simulink model "controller_main"  (R2025a)
settings: Solver=VariableStepAuto  StartTime=0.0  StopTime=inf  RelTol=1e-3
model workspace (MAT data in the model file):
  input_force = 1000
  input_moment = 300
  input_radius = 1
  input_theta = 0.785398163397
settings Model: Creator=TAK  LastModifiedBy=TAK

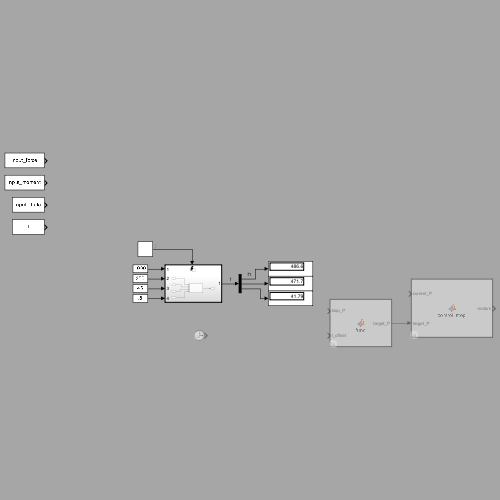
[thumbnail: Simulink's stored preview of the top-level diagram]
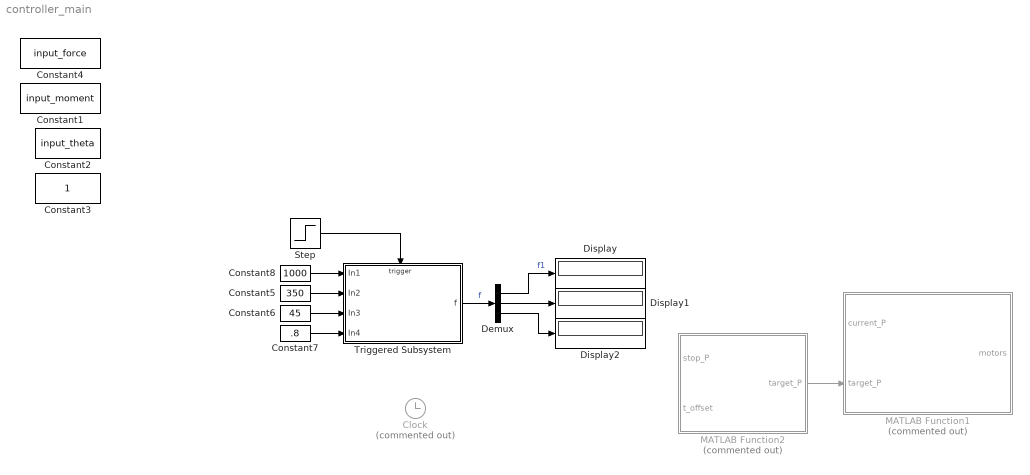
== system controller_main ==
  Clock : Clock  Commented=on
  Constant1 : Constant  Value=input_moment
  Constant2 : Constant  Value=input_theta
  Constant3 : Constant
  Constant4 : Constant  Value=input_force
  Constant5 : Constant  Value=350
  Constant6 : Constant  Value=45
  Constant7 : Constant  Value=.8
  Constant8 : Constant  Value=1000
  Demux : Demux  Outputs=3
  Display : Display
  Display1 : Display
  Display2 : Display
  MATLAB Function1 : MATLAB Function  Commented=on  TreatAsAtomicUnit=on
  MATLAB Function2 : MATLAB Function  Commented=on  TreatAsAtomicUnit=on
  Step : Step  Time=0  SampleTime=0
  Triggered Subsystem : Subsystem  TreatAsAtomicUnit=on
  wires:
  MATLAB Function2/1(target_P) -> MATLAB Function1/2(target_P)
  Step/1 -> Triggered Subsystem/Trigger
  Triggered Subsystem/1(f) -> Demux/1  "f"
  Demux/3 -> Display2/1
  Demux/1 -> Display/1  "f1"
  Demux/2 -> Display1/1
  Constant8/1 -> Triggered Subsystem/1(In1)
  Constant5/1 -> Triggered Subsystem/2(In2)
  Constant6/1 -> Triggered Subsystem/3(In3)
  Constant7/1 -> Triggered Subsystem/4(In4)

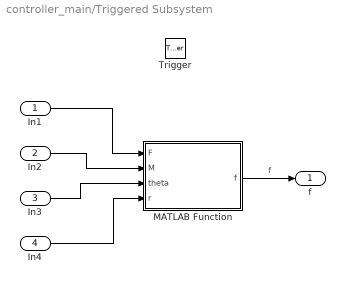
== system controller_main/Triggered Subsystem ==
  In1 : Inport
  In2 : Inport  Port=2
  In3 : Inport  Port=3
  In4 : Inport  Port=4
  Trigger : TriggerPort  VariantControl=(inherit)  InitialTriggerSignalState=zero
  MATLAB Function : MATLAB Function  TreatAsAtomicUnit=on
  f : Outport
  wires:
  In1/1 -> MATLAB Function/1(F)
  In4/1 -> MATLAB Function/4(r)
  In3/1 -> MATLAB Function/3(theta)
  In2/1 -> MATLAB Function/2(M)
  MATLAB Function/1(f) -> f/1  "f"

== matlab function controller_main/MATLAB Function1 ==
  data: current_P input; motors output; target_P input
function motors  = control_step(current_P, target_P)
    motors = control_step(current_P, target_P);
end

== matlab function controller_main/Triggered Subsystem/MATLAB Function ==
  data: F input; f output; M input; theta input; r input
function f   = calc_forces(F, M, theta, r)
    % F       compressive force [N]
    % M       bending moment [Nm]
    % theta   angle moment is applied at [rad]
    % r       radius of actuators [m]
    f = [0 0 0];
    f(1) = 1/3 * (F + 2*M*cos(theta)/r);
    f(2) = 1/3 * (F + (sqrt(3)*M*sin(theta) - M*cos(theta))/r);
    f(3) = 1/3 * (F + (-sqrt(3)*M*sin(theta) - M*cos(theta))/r);
end

== matlab function controller_main/MATLAB Function2 ==
  data: stop_P input; target_P output; t_offset input
function target_P  = func(stop_P, t_offset)

y = u;
